simulink model "T_TEM_OCV"  (R2015a)
settings: Solver=ode3  StartTime=0.0  StopTime=159  FixedStep=1  RelTol=1e-3
values from neighbouring files (symbols this model uses):
  I = 0    [TEM_OCV.m]    (also in matched.mat = )
libraries: LU_TEG x1
settings Model: Creator=lansong7  LastModifiedBy=ttsl6

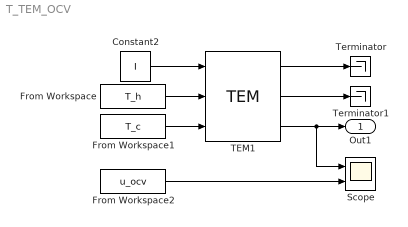
== system T_TEM_OCV ==
  Constant2 : Constant  Value=I
  From Workspace : FromWorkspace  VariableName=T_h  SampleTime=0
  From Workspace1 : FromWorkspace  VariableName=T_c  SampleTime=0
  From Workspace2 : FromWorkspace  VariableName=u_ocv  SampleTime=0
  Scope : Scope  NumInputPorts=2
      settings: TimeRange=159  YMin=300~0  YMax=380~7
  TEM1 : LU_TEG/TEM  l=l  l_cw=l_cw  f=f  a=a  n=n  Tune_tr=Tune_tr  ce1=ce1  ce2=ce2  ct1=ct1  ct2=ct2
  Terminator : Terminator
  Terminator1 : Terminator
  Out1 : Outport
  wires:
  From Workspace/1 -> TEM1/2
  From Workspace1/1 -> TEM1/3
  Constant2/1 -> TEM1/1
  TEM1/3 -> Scope/1, Out1/1
  TEM1/2 -> Terminator1/1
  TEM1/1 -> Terminator/1
  From Workspace2/1 -> Scope/2
